simulink library "lib_TCML"  (R2015a)
settings: Solver=ode45  StartTime=0.0  StopTime=10.0  RelTol=1e-3
libraries: simulink x5
(part 5 of 7)

== system lib_TCML/Dynamic Tip Clearance/Case Deformation/Deformation1/Thermal Expansion 1D Elastic ==
  Previous/Reference Length [Lo] : Inport
  Previous/Reference Temperature [To] : Inport  Port=2
  Current Temperature [Tf] : Inport  Port=3
  Add : Sum  Inputs=+-
  Add1 : Sum
  MATLAB Function : MATLAB Function  TreatAsAtomicUnit=on
  Mass Flow Rate on Inner Surface1 : Constant  Value=TempDependence_M
  Mass Flow Rate on Inner Surface2 : Constant  Value=T_data_M
  Mass Flow Rate on Inner Surface3 : Constant  Value=alpha_data_M
  Mass Flow Rate on Inner Surface4 : Constant  Value=alpha_M
  Mass Flow Rate on Inner Surface6 : Constant  Value=BN_M
  Memory : Memory  X0=zeros(1,7)  InheritSampleTime=on
  Product : Product  Inputs=***
  Switch : Switch  Criteria=u2 > Threshold
  Current Length [L] : Outport
  wires:
  Previous/Reference Length [Lo]/1 -> Product/2, Add1/2, MATLAB Function/3(Lo)
  Previous/Reference Temperature [To]/1 -> MATLAB Function/4(To), Add/2
  Current Temperature [Tf]/1 -> MATLAB Function/5(Tf), Add/1
  Mass Flow Rate on Inner Surface6/1 -> MATLAB Function/7(BN)
  MATLAB Function/1(L) -> Switch/1
  Memory/1 -> MATLAB Function/6(Erro)
  MATLAB Function/2(Err) -> Memory/1
  Mass Flow Rate on Inner Surface1/1 -> Switch/2
  Mass Flow Rate on Inner Surface2/1 -> MATLAB Function/1(T_data)
  Mass Flow Rate on Inner Surface3/1 -> MATLAB Function/2(alpha_data)
  Add/1 -> Product/1
  Mass Flow Rate on Inner Surface4/1 -> Product/3
  Switch/1 -> Current Length [L]/1
  Product/1 -> Add1/1
  Add1/1 -> Switch/3

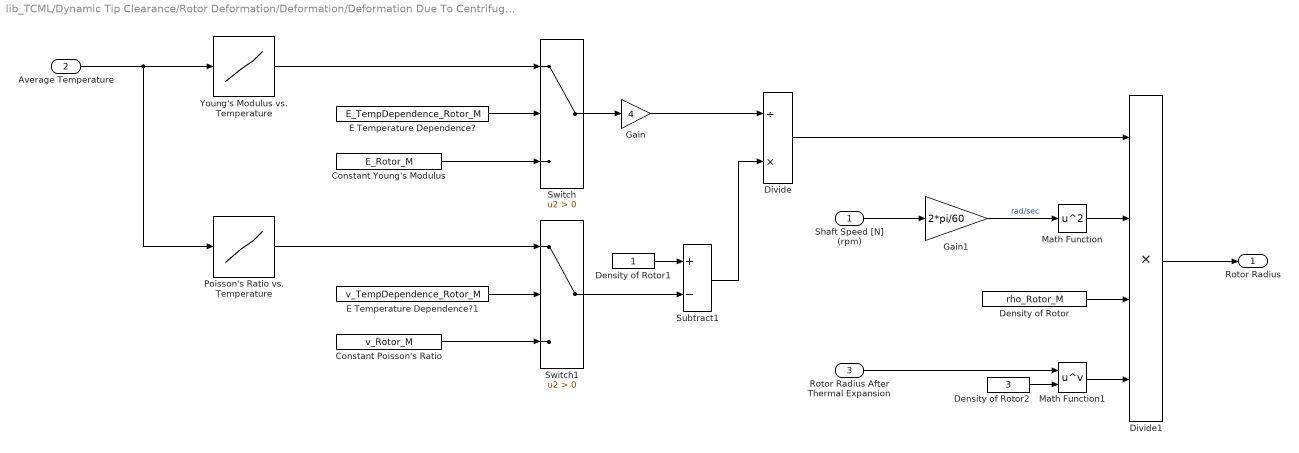
== system lib_TCML/Dynamic Tip Clearance/Rotor Deformation/Deformation/Deformation Due To Centrifugal Forces ==
  Shaft Speed [N] (rpm) : Inport
  Average Temperature : Inport  Port=2
  Rotor Radius After Thermal Expansion : Inport  Port=3
  Constant Poisson's Ratio : Constant  Value=v_Rotor_M
  Constant Young's Modulus : Constant  Value=E_Rotor_M
  Density of Rotor : Constant  Value=rho_Rotor_M
  Density of Rotor1 : Constant
  Density of Rotor2 : Constant  Value=3
  Divide : Product  Inputs=/*
  Divide1 : Product  Inputs=****
  E Temperature Dependence? : Constant  Value=E_TempDependence_Rotor_M
  E Temperature Dependence?1 : Constant  Value=v_TempDependence_Rotor_M
  Gain : Gain  Gain=4
  Gain1 : Gain  Gain=2*pi/60
  Math Function : Math  Operator=square  SaturateOnIntegerOverflow=on
  Math Function1 : Math  Operator=pow  SaturateOnIntegerOverflow=on
  Poisson's Ratio vs. Temperature : Lookup_n-D  NumberOfTableDimensions=1  BreakpointsForDimension1=Tv_Rotor_Data_M  Table=v_Rotor_Data_M  InternalRulePriority=Speed  RndMeth=Simplest  InputSameDT=on
  Subtract1 : Sum  Inputs=+-
  Switch : Switch  Criteria=u2 > Threshold
  Switch1 : Switch  Criteria=u2 > Threshold
  Young's Modulus vs. Temperature : Lookup_n-D  NumberOfTableDimensions=1  BreakpointsForDimension1=TE_Rotor_Data_M  Table=E_Rotor_Data_M  InternalRulePriority=Speed  RndMeth=Simplest  InputSameDT=on
  Rotor Radius : Outport
  wires:
  Constant Poisson's Ratio/1 -> Switch1/3
  Young's Modulus vs. Temperature/1 -> Switch/1
  Poisson's Ratio vs. Temperature/1 -> Switch1/1
  E Temperature Dependence?1/1 -> Switch1/2
  Switch/1 -> Gain/1
  Density of Rotor1/1 -> Subtract1/1
  Constant Young's Modulus/1 -> Switch/3
  Divide/1 -> Divide1/1
  Switch1/1 -> Subtract1/2
  Subtract1/1 -> Divide/2
  Gain/1 -> Divide/1
  Gain1/1 -> Math Function/1  "rad/sec"
  Density of Rotor/1 -> Divide1/3
  E Temperature Dependence?/1 -> Switch/2
  Math Function1/1 -> Divide1/4
  Math Function/1 -> Divide1/2
  Shaft Speed [N] (rpm)/1 -> Gain1/1
  Divide1/1 -> Rotor Radius/1
  Density of Rotor2/1 -> Math Function1/2
  Average Temperature/1 -> Poisson's Ratio vs. Temperature/1, Young's Modulus vs. Temperature/1
  Rotor Radius After Thermal Expansion/1 -> Math Function1/1

== system lib_TCML/Dynamic Tip Clearance/Rotor Deformation/Deformation/Deformation Due To Thermal Expansion ==
  Average Rotor Temperature : Inport
  Memory1 : Memory  X0=mean(T0_Rotor_M)
  Memory2 : Memory  X0=Ro_Rotor_M
  Thermal Expansion 1D Elastic : Subsystem  mask(TSAT: Thermal Expansion Library Block){TempDependence_M=on, alpha_M=alpha_Rotor_M, T_data_M=Talpha_Rotor_Data_M, alpha_data_M=alpha_Rotor_Data_M, BN_M=double(gcb)}
      mask prompts: TempDependence_M "TempDependence_M - Temperature dependence of the thermal expansion coefficient (unchecked - constant, checked - temperature dependent)"; alpha_M "alpha_M - Constant thermal expansion coefficient"; T_data_M "T_data_M - Temperature array (nx1)"; alpha_data_M "alpha_data_M - Thermal expansion coefficient array (nx1)"; BN_M "Block Name"
      mask help:
      | This function calculates the length or radius of a structure that has expanded or contracted due to thermal expansion. The block accepts the previous/reference length (Lo), previous/reference temperature (To), and current temperature (Tf) as its inputs. The user has the option to specify a constant thermal expansion coefficient or to incorporate temperature dependence by providing data that correlates the thermal expansion coefficient with temperature.
      |
      | This block is capable of accepting various units but it is important that the units be consistent across all inputs and parameters. For details on this block, see the block help menu.
      mask init:
      | %set default parameters if they are not being used
      | if TempDependence_M == 0
      |     T_data_M = [0 5000];
      |     alpha_data_M = [10e-6 10e-6];
      | elseif TempDependence_M == 1
      |     alpha_M = 10e-6;
      | end
      mask Help: web(which('Deformation_TSAT_ThermExp1DElastic.html'),'-helpbrowser')
      mask Callback TempDependence_M:
      | MSK_SEC_Enables_TSAT('TempDependence_M',2,'dis')
      | MSK_SEC_Enables_TSAT('TempDependence_M',[3 4],'en')
  Rotor Radius after Thermal Expansion : Outport
  wires:
  Average Rotor Temperature/1 -> Thermal Expansion 1D Elastic/3(Current Temperature [Tf]), Memory1/1
  Memory2/1 -> Thermal Expansion 1D Elastic/1(Previous/Reference Length [Lo])
  Memory1/1 -> Thermal Expansion 1D Elastic/2(Previous/Reference Temperature [To])
  Thermal Expansion 1D Elastic/1(Current Length [L]) -> Memory2/1, Rotor Radius after Thermal Expansion/1

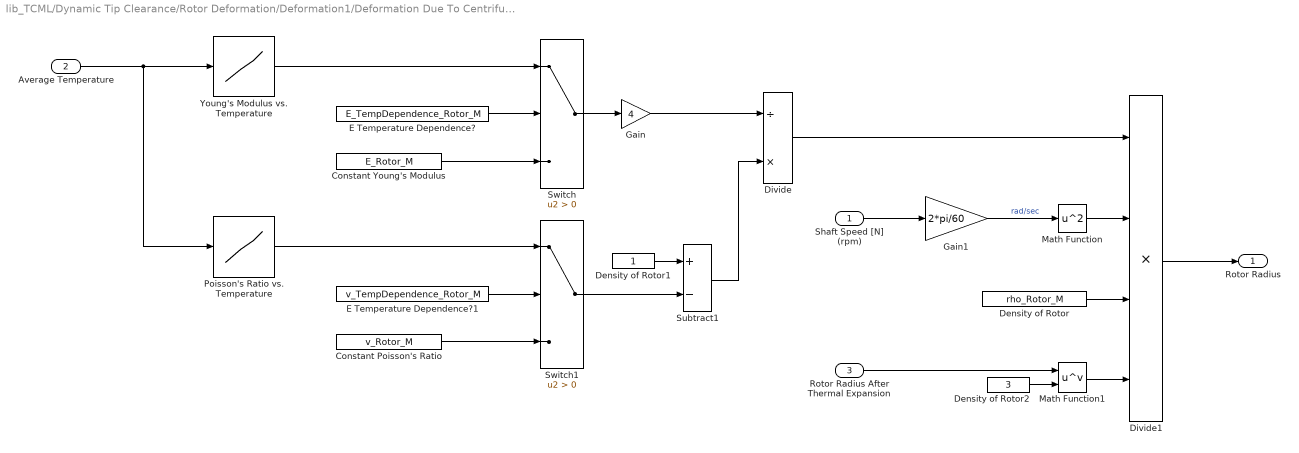
== system lib_TCML/Dynamic Tip Clearance/Rotor Deformation/Deformation1/Deformation Due To Centrifugal Forces ==
  Shaft Speed [N] (rpm) : Inport
  Average Temperature : Inport  Port=2
  Rotor Radius After Thermal Expansion : Inport  Port=3
  Constant Poisson's Ratio : Constant  Value=v_Rotor_M
  Constant Young's Modulus : Constant  Value=E_Rotor_M
  Density of Rotor : Constant  Value=rho_Rotor_M
  Density of Rotor1 : Constant
  Density of Rotor2 : Constant  Value=3
  Divide : Product  Inputs=/*
  Divide1 : Product  Inputs=****
  E Temperature Dependence? : Constant  Value=E_TempDependence_Rotor_M
  E Temperature Dependence?1 : Constant  Value=v_TempDependence_Rotor_M
  Gain : Gain  Gain=4
  Gain1 : Gain  Gain=2*pi/60
  Math Function : Math  Operator=square  SaturateOnIntegerOverflow=on
  Math Function1 : Math  Operator=pow  SaturateOnIntegerOverflow=on
  Poisson's Ratio vs. Temperature : Lookup_n-D  NumberOfTableDimensions=1  BreakpointsForDimension1=Tv_Rotor_Data_M  Table=v_Rotor_Data_M  InternalRulePriority=Speed  RndMeth=Simplest  InputSameDT=on
  Subtract1 : Sum  Inputs=+-
  Switch : Switch  Criteria=u2 > Threshold
  Switch1 : Switch  Criteria=u2 > Threshold
  Young's Modulus vs. Temperature : Lookup_n-D  NumberOfTableDimensions=1  BreakpointsForDimension1=TE_Rotor_Data_M  Table=E_Rotor_Data_M  InternalRulePriority=Speed  RndMeth=Simplest  InputSameDT=on
  Rotor Radius : Outport
  wires:
  Rotor Radius After Thermal Expansion/1 -> Math Function1/1
  Average Temperature/1 -> Young's Modulus vs. Temperature/1, Poisson's Ratio vs. Temperature/1
  Density of Rotor2/1 -> Math Function1/2
  Divide1/1 -> Rotor Radius/1
  Shaft Speed [N] (rpm)/1 -> Gain1/1
  Math Function/1 -> Divide1/2
  Math Function1/1 -> Divide1/4
  E Temperature Dependence?/1 -> Switch/2
  Density of Rotor/1 -> Divide1/3
  Gain1/1 -> Math Function/1  "rad/sec"
  Gain/1 -> Divide/1
  Subtract1/1 -> Divide/2
  Switch1/1 -> Subtract1/2
  Divide/1 -> Divide1/1
  Constant Young's Modulus/1 -> Switch/3
  Density of Rotor1/1 -> Subtract1/1
  Switch/1 -> Gain/1
  E Temperature Dependence?1/1 -> Switch1/2
  Poisson's Ratio vs. Temperature/1 -> Switch1/1
  Young's Modulus vs. Temperature/1 -> Switch/1
  Constant Poisson's Ratio/1 -> Switch1/3

== system lib_TCML/Dynamic Tip Clearance/Rotor Deformation/Deformation1/Deformation Due To Thermal Expansion ==
  Average Rotor Temperature : Inport
  Memory1 : Memory  X0=mean(T0_Rotor_M)
  Memory2 : Memory  X0=Ro_Rotor_M
  Thermal Expansion 1D Elastic : Subsystem  mask(TSAT: Thermal Expansion Library Block){TempDependence_M=on, alpha_M=alpha_Rotor_M, T_data_M=Talpha_Rotor_Data_M, alpha_data_M=alpha_Rotor_Data_M, BN_M=double(gcb)}
      mask prompts: TempDependence_M "TempDependence_M - Temperature dependence of the thermal expansion coefficient (unchecked - constant, checked - temperature dependent)"; alpha_M "alpha_M - Constant thermal expansion coefficient"; T_data_M "T_data_M - Temperature array (nx1)"; alpha_data_M "alpha_data_M - Thermal expansion coefficient array (nx1)"; BN_M "Block Name"
      mask help:
      | This function calculates the length or radius of a structure that has expanded or contracted due to thermal expansion. The block accepts the previous/reference length (Lo), previous/reference temperature (To), and current temperature (Tf) as its inputs. The user has the option to specify a constant thermal expansion coefficient or to incorporate temperature dependence by providing data that correlates the thermal expansion coefficient with temperature.
      |
      | This block is capable of accepting various units but it is important that the units be consistent across all inputs and parameters. For details on this block, see the block help menu.
      mask init:
      | %set default parameters if they are not being used
      | if TempDependence_M == 0
      |     T_data_M = [0 5000];
      |     alpha_data_M = [10e-6 10e-6];
      | elseif TempDependence_M == 1
      |     alpha_M = 10e-6;
      | end
      mask Help: web(which('Deformation_TSAT_ThermExp1DElastic.html'),'-helpbrowser')
      mask Callback TempDependence_M:
      | MSK_SEC_Enables_TSAT('TempDependence_M',2,'dis')
      | MSK_SEC_Enables_TSAT('TempDependence_M',[3 4],'en')
  Rotor Radius after Thermal Expansion : Outport
  wires:
  Thermal Expansion 1D Elastic/1(Current Length [L]) -> Rotor Radius after Thermal Expansion/1, Memory2/1
  Memory1/1 -> Thermal Expansion 1D Elastic/2(Previous/Reference Temperature [To])
  Memory2/1 -> Thermal Expansion 1D Elastic/1(Previous/Reference Length [Lo])
  Average Rotor Temperature/1 -> Memory1/1, Thermal Expansion 1D Elastic/3(Current Temperature [Tf])

== system lib_TCML/Steady-State Tip Clearance/Blade Deformation/Deformation/Deformation Due To Centrifugal Forces ==
  Shaft Speed [N] (rpm) : Inport
  Average Temperature : Inport  Port=2
  Blade Length After Thermal Expansion : Inport  Port=3
  Rotor Outer Radius : Inport  Port=4
  Add : Sum
  Constant Young's Modulus : Constant  Value=E_Blade_M
  Density of Rotor : Constant  Value=rho_Blade_M
  Density of Rotor1 : Constant
  Divide : Product  Inputs=/*
  Divide1 : Product  Inputs=****
  Divide2 : Product  Inputs=**
  E Temperature Dependence? : Constant  Value=E_TempDependence_Blade_M
  Gain1 : Gain  Gain=2*pi/60
  Math Function : Math  Operator=square  SaturateOnIntegerOverflow=on
  Math Function2 : Math  Operator=square  SaturateOnIntegerOverflow=on
  Switch : Switch  Criteria=u2 > Threshold
  Young's Modulus vs. Temperature : Lookup_n-D  NumberOfTableDimensions=1  BreakpointsForDimension1=TE_Blade_Data_M  Table=E_Blade_Data_M  InternalRulePriority=Speed  RndMeth=Simplest  InputSameDT=on
  Blade Length : Outport
  wires:
  Young's Modulus vs. Temperature/1 -> Switch/1
  Density of Rotor1/1 -> Divide/2
  Constant Young's Modulus/1 -> Switch/3
  Divide/1 -> Divide1/1
  Switch/1 -> Divide/1
  Gain1/1 -> Math Function/1  "rad/sec"
  Density of Rotor/1 -> Divide1/3
  E Temperature Dependence?/1 -> Switch/2
  Math Function/1 -> Divide1/2
  Shaft Speed [N] (rpm)/1 -> Gain1/1
  Divide1/1 -> Blade Length/1
  Average Temperature/1 -> Young's Modulus vs. Temperature/1
  Blade Length After Thermal Expansion/1 -> Add/2, Math Function2/1
  Rotor Outer Radius/1 -> Add/1
  Add/1 -> Divide2/1
  Math Function2/1 -> Divide2/2
  Divide2/1 -> Divide1/4

== system lib_TCML/Steady-State Tip Clearance/Blade Deformation/Deformation/Deformation Due To Thermal Expansion ==
  Average Rotor Temperature : Inport
  Memory1 : Memory  X0=T0_Blade_M
  Memory2 : Memory  X0=L_Blade_M
  Thermal Expansion 1D Elastic : Subsystem  mask(TSAT: Thermal Expansion Library Block){TempDependence_M=on, alpha_M=alpha_Blade_M, T_data_M=Talpha_Blade_Data_M, alpha_data_M=alpha_Blade_Data_M, BN_M=double(gcb)}
      mask prompts: TempDependence_M "TempDependence_M - Temperature dependence of the thermal expansion coefficient (unchecked - constant, checked - temperature dependent)"; alpha_M "alpha_M - Constant thermal expansion coefficient"; T_data_M "T_data_M - Temperature array (nx1)"; alpha_data_M "alpha_data_M - Thermal expansion coefficient array (nx1)"; BN_M "Block Name"
      mask help:
      | This function calculates the length or radius of a structure that has expanded or contracted due to thermal expansion. The block accepts the previous/reference length (Lo), previous/reference temperature (To), and current temperature (Tf) as its inputs. The user has the option to specify a constant thermal expansion coefficient or to incorporate temperature dependence by providing data that correlates the thermal expansion coefficient with temperature.
      |
      | This block is capable of accepting various units but it is important that the units be consistent across all inputs and parameters. For details on this block, see the block help menu.
      mask init:
      | %set default parameters if they are not being used
      | if TempDependence_M == 0
      |     T_data_M = [0 5000];
      |     alpha_data_M = [10e-6 10e-6];
      | elseif TempDependence_M == 1
      |     alpha_M = 10e-6;
      | end
      mask Help: web(which('Deformation_TSAT_ThermExp1DElastic.html'),'-helpbrowser')
      mask Callback TempDependence_M:
      | MSK_SEC_Enables_TSAT('TempDependence_M',2,'dis')
      | MSK_SEC_Enables_TSAT('TempDependence_M',[3 4],'en')
  Blade Length after Thermal Expansion : Outport
  wires:
  Average Rotor Temperature/1 -> Thermal Expansion 1D Elastic/3(Current Temperature [Tf]), Memory1/1
  Memory2/1 -> Thermal Expansion 1D Elastic/1(Previous/Reference Length [Lo])
  Memory1/1 -> Thermal Expansion 1D Elastic/2(Previous/Reference Temperature [To])
  Thermal Expansion 1D Elastic/1(Current Length [L]) -> Memory2/1, Blade Length after Thermal Expansion/1

== system lib_TCML/Steady-State Tip Clearance/Case Deformation/Deformation/Thermal Expansion 1D Elastic ==
  Previous/Reference Length [Lo] : Inport
  Previous/Reference Temperature [To] : Inport  Port=2
  Current Temperature [Tf] : Inport  Port=3
  Add : Sum  Inputs=+-
  Add1 : Sum
  MATLAB Function : MATLAB Function  TreatAsAtomicUnit=on
  Mass Flow Rate on Inner Surface1 : Constant  Value=TempDependence_M
  Mass Flow Rate on Inner Surface2 : Constant  Value=T_data_M
  Mass Flow Rate on Inner Surface3 : Constant  Value=alpha_data_M
  Mass Flow Rate on Inner Surface4 : Constant  Value=alpha_M
  Mass Flow Rate on Inner Surface6 : Constant  Value=BN_M
  Memory : Memory  X0=zeros(1,7)  InheritSampleTime=on
  Product : Product  Inputs=***
  Switch : Switch  Criteria=u2 > Threshold
  Current Length [L] : Outport
  wires:
  Previous/Reference Length [Lo]/1 -> Product/2, Add1/2, MATLAB Function/3(Lo)
  Previous/Reference Temperature [To]/1 -> MATLAB Function/4(To), Add/2
  Current Temperature [Tf]/1 -> MATLAB Function/5(Tf), Add/1
  Mass Flow Rate on Inner Surface6/1 -> MATLAB Function/7(BN)
  MATLAB Function/1(L) -> Switch/1
  Memory/1 -> MATLAB Function/6(Erro)
  MATLAB Function/2(Err) -> Memory/1
  Mass Flow Rate on Inner Surface1/1 -> Switch/2
  Mass Flow Rate on Inner Surface2/1 -> MATLAB Function/1(T_data)
  Mass Flow Rate on Inner Surface3/1 -> MATLAB Function/2(alpha_data)
  Add/1 -> Product/1
  Mass Flow Rate on Inner Surface4/1 -> Product/3
  Switch/1 -> Current Length [L]/1
  Product/1 -> Add1/1
  Add1/1 -> Switch/3

== system lib_TCML/Steady-State Tip Clearance/Case Deformation/Deformation1/Thermal Expansion 1D Elastic ==
  Previous/Reference Length [Lo] : Inport
  Previous/Reference Temperature [To] : Inport  Port=2
  Current Temperature [Tf] : Inport  Port=3
  Add : Sum  Inputs=+-
  Add1 : Sum
  MATLAB Function : MATLAB Function  TreatAsAtomicUnit=on
  Mass Flow Rate on Inner Surface1 : Constant  Value=TempDependence_M
  Mass Flow Rate on Inner Surface2 : Constant  Value=T_data_M
  Mass Flow Rate on Inner Surface3 : Constant  Value=alpha_data_M
  Mass Flow Rate on Inner Surface4 : Constant  Value=alpha_M
  Mass Flow Rate on Inner Surface6 : Constant  Value=BN_M
  Memory : Memory  X0=zeros(1,7)  InheritSampleTime=on
  Product : Product  Inputs=***
  Switch : Switch  Criteria=u2 > Threshold
  Current Length [L] : Outport
  wires:
  Add1/1 -> Switch/3
  Product/1 -> Add1/1
  Switch/1 -> Current Length [L]/1
  Mass Flow Rate on Inner Surface4/1 -> Product/3
  Add/1 -> Product/1
  Mass Flow Rate on Inner Surface3/1 -> MATLAB Function/2(alpha_data)
  Mass Flow Rate on Inner Surface2/1 -> MATLAB Function/1(T_data)
  Mass Flow Rate on Inner Surface1/1 -> Switch/2
  MATLAB Function/2(Err) -> Memory/1
  Memory/1 -> MATLAB Function/6(Erro)
  MATLAB Function/1(L) -> Switch/1
  Mass Flow Rate on Inner Surface6/1 -> MATLAB Function/7(BN)
  Current Temperature [Tf]/1 -> Add/1, MATLAB Function/5(Tf)
  Previous/Reference Temperature [To]/1 -> Add/2, MATLAB Function/4(To)
  Previous/Reference Length [Lo]/1 -> MATLAB Function/3(Lo), Add1/2, Product/2

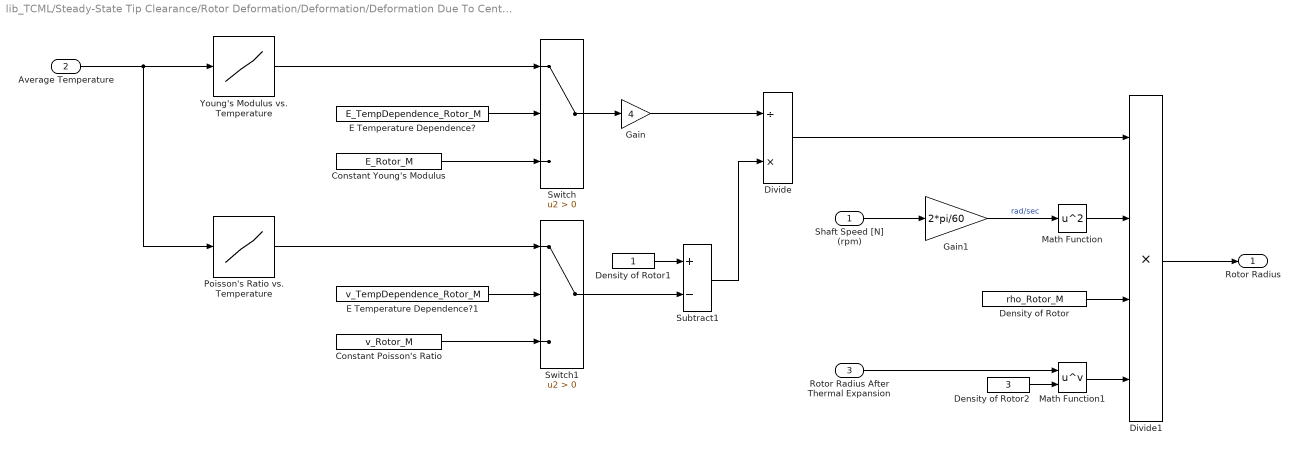
== system lib_TCML/Steady-State Tip Clearance/Rotor Deformation/Deformation/Deformation Due To Centrifugal Forces ==
  Shaft Speed [N] (rpm) : Inport
  Average Temperature : Inport  Port=2
  Rotor Radius After Thermal Expansion : Inport  Port=3
  Constant Poisson's Ratio : Constant  Value=v_Rotor_M
  Constant Young's Modulus : Constant  Value=E_Rotor_M
  Density of Rotor : Constant  Value=rho_Rotor_M
  Density of Rotor1 : Constant
  Density of Rotor2 : Constant  Value=3
  Divide : Product  Inputs=/*
  Divide1 : Product  Inputs=****
  E Temperature Dependence? : Constant  Value=E_TempDependence_Rotor_M
  E Temperature Dependence?1 : Constant  Value=v_TempDependence_Rotor_M
  Gain : Gain  Gain=4
  Gain1 : Gain  Gain=2*pi/60
  Math Function : Math  Operator=square  SaturateOnIntegerOverflow=on
  Math Function1 : Math  Operator=pow  SaturateOnIntegerOverflow=on
  Poisson's Ratio vs. Temperature : Lookup_n-D  NumberOfTableDimensions=1  BreakpointsForDimension1=Tv_Rotor_Data_M  Table=v_Rotor_Data_M  InternalRulePriority=Speed  RndMeth=Simplest  InputSameDT=on
  Subtract1 : Sum  Inputs=+-
  Switch : Switch  Criteria=u2 > Threshold
  Switch1 : Switch  Criteria=u2 > Threshold
  Young's Modulus vs. Temperature : Lookup_n-D  NumberOfTableDimensions=1  BreakpointsForDimension1=TE_Rotor_Data_M  Table=E_Rotor_Data_M  InternalRulePriority=Speed  RndMeth=Simplest  InputSameDT=on
  Rotor Radius : Outport
  wires:
  Constant Poisson's Ratio/1 -> Switch1/3
  Young's Modulus vs. Temperature/1 -> Switch/1
  Poisson's Ratio vs. Temperature/1 -> Switch1/1
  E Temperature Dependence?1/1 -> Switch1/2
  Switch/1 -> Gain/1
  Density of Rotor1/1 -> Subtract1/1
  Constant Young's Modulus/1 -> Switch/3
  Divide/1 -> Divide1/1
  Switch1/1 -> Subtract1/2
  Subtract1/1 -> Divide/2
  Gain/1 -> Divide/1
  Gain1/1 -> Math Function/1  "rad/sec"
  Density of Rotor/1 -> Divide1/3
  E Temperature Dependence?/1 -> Switch/2
  Math Function1/1 -> Divide1/4
  Math Function/1 -> Divide1/2
  Shaft Speed [N] (rpm)/1 -> Gain1/1
  Divide1/1 -> Rotor Radius/1
  Density of Rotor2/1 -> Math Function1/2
  Average Temperature/1 -> Poisson's Ratio vs. Temperature/1, Young's Modulus vs. Temperature/1
  Rotor Radius After Thermal Expansion/1 -> Math Function1/1

== system lib_TCML/Steady-State Tip Clearance/Rotor Deformation/Deformation/Deformation Due To Thermal Expansion ==
  Average Rotor Temperature : Inport
  Memory1 : Memory  X0=mean(T0_Rotor_M)
  Memory2 : Memory  X0=Ro_Rotor_M
  Thermal Expansion 1D Elastic : Subsystem  mask(TSAT: Thermal Expansion Library Block){TempDependence_M=on, alpha_M=alpha_Rotor_M, T_data_M=Talpha_Rotor_Data_M, alpha_data_M=alpha_Rotor_Data_M, BN_M=double(gcb)}
      mask prompts: TempDependence_M "TempDependence_M - Temperature dependence of the thermal expansion coefficient (unchecked - constant, checked - temperature dependent)"; alpha_M "alpha_M - Constant thermal expansion coefficient"; T_data_M "T_data_M - Temperature array (nx1)"; alpha_data_M "alpha_data_M - Thermal expansion coefficient array (nx1)"; BN_M "Block Name"
      mask help:
      | This function calculates the length or radius of a structure that has expanded or contracted due to thermal expansion. The block accepts the previous/reference length (Lo), previous/reference temperature (To), and current temperature (Tf) as its inputs. The user has the option to specify a constant thermal expansion coefficient or to incorporate temperature dependence by providing data that correlates the thermal expansion coefficient with temperature.
      |
      | This block is capable of accepting various units but it is important that the units be consistent across all inputs and parameters. For details on this block, see the block help menu.
      mask init:
      | %set default parameters if they are not being used
      | if TempDependence_M == 0
      |     T_data_M = [0 5000];
      |     alpha_data_M = [10e-6 10e-6];
      | elseif TempDependence_M == 1
      |     alpha_M = 10e-6;
      | end
      mask Help: web(which('Deformation_TSAT_ThermExp1DElastic.html'),'-helpbrowser')
      mask Callback TempDependence_M:
      | MSK_SEC_Enables_TSAT('TempDependence_M',2,'dis')
      | MSK_SEC_Enables_TSAT('TempDependence_M',[3 4],'en')
  Rotor Radius after Thermal Expansion : Outport
  wires:
  Average Rotor Temperature/1 -> Thermal Expansion 1D Elastic/3(Current Temperature [Tf]), Memory1/1
  Memory2/1 -> Thermal Expansion 1D Elastic/1(Previous/Reference Length [Lo])
  Memory1/1 -> Thermal Expansion 1D Elastic/2(Previous/Reference Temperature [To])
  Thermal Expansion 1D Elastic/1(Current Length [L]) -> Memory2/1, Rotor Radius after Thermal Expansion/1

== system lib_TCML/Dynamic Tip Clearance/Blade Deformation/Deformation/Deformation Due To Thermal Expansion/Thermal Expansion 1D Elastic ==
  Previous/Reference Length [Lo] : Inport
  Previous/Reference Temperature [To] : Inport  Port=2
  Current Temperature [Tf] : Inport  Port=3
  Add : Sum  Inputs=+-
  Add1 : Sum
  MATLAB Function : MATLAB Function  TreatAsAtomicUnit=on
  Mass Flow Rate on Inner Surface1 : Constant  Value=TempDependence_M
  Mass Flow Rate on Inner Surface2 : Constant  Value=T_data_M
  Mass Flow Rate on Inner Surface3 : Constant  Value=alpha_data_M
  Mass Flow Rate on Inner Surface4 : Constant  Value=alpha_M
  Mass Flow Rate on Inner Surface6 : Constant  Value=BN_M
  Memory : Memory  X0=zeros(1,7)  InheritSampleTime=on
  Product : Product  Inputs=***
  Switch : Switch  Criteria=u2 > Threshold
  Current Length [L] : Outport
  wires:
  Previous/Reference Length [Lo]/1 -> Product/2, Add1/2, MATLAB Function/3(Lo)
  Previous/Reference Temperature [To]/1 -> MATLAB Function/4(To), Add/2
  Current Temperature [Tf]/1 -> MATLAB Function/5(Tf), Add/1
  Mass Flow Rate on Inner Surface6/1 -> MATLAB Function/7(BN)
  MATLAB Function/1(L) -> Switch/1
  Memory/1 -> MATLAB Function/6(Erro)
  MATLAB Function/2(Err) -> Memory/1
  Mass Flow Rate on Inner Surface1/1 -> Switch/2
  Mass Flow Rate on Inner Surface2/1 -> MATLAB Function/1(T_data)
  Mass Flow Rate on Inner Surface3/1 -> MATLAB Function/2(alpha_data)
  Add/1 -> Product/1
  Mass Flow Rate on Inner Surface4/1 -> Product/3
  Switch/1 -> Current Length [L]/1
  Product/1 -> Add1/1
  Add1/1 -> Switch/3

== system lib_TCML/Dynamic Tip Clearance/Blade Deformation/Deformation1/Deformation Due To Thermal Expansion/Thermal Expansion 1D Elastic ==
  Previous/Reference Length [Lo] : Inport
  Previous/Reference Temperature [To] : Inport  Port=2
  Current Temperature [Tf] : Inport  Port=3
  Add : Sum  Inputs=+-
  Add1 : Sum
  MATLAB Function : MATLAB Function  TreatAsAtomicUnit=on
  Mass Flow Rate on Inner Surface1 : Constant  Value=TempDependence_M
  Mass Flow Rate on Inner Surface2 : Constant  Value=T_data_M
  Mass Flow Rate on Inner Surface3 : Constant  Value=alpha_data_M
  Mass Flow Rate on Inner Surface4 : Constant  Value=alpha_M
  Mass Flow Rate on Inner Surface6 : Constant  Value=BN_M
  Memory : Memory  X0=zeros(1,7)  InheritSampleTime=on
  Product : Product  Inputs=***
  Switch : Switch  Criteria=u2 > Threshold
  Current Length [L] : Outport
  wires:
  Previous/Reference Length [Lo]/1 -> Product/2, Add1/2, MATLAB Function/3(Lo)
  Previous/Reference Temperature [To]/1 -> MATLAB Function/4(To), Add/2
  Current Temperature [Tf]/1 -> MATLAB Function/5(Tf), Add/1
  Mass Flow Rate on Inner Surface6/1 -> MATLAB Function/7(BN)
  MATLAB Function/1(L) -> Switch/1
  Memory/1 -> MATLAB Function/6(Erro)
  MATLAB Function/2(Err) -> Memory/1
  Mass Flow Rate on Inner Surface1/1 -> Switch/2
  Mass Flow Rate on Inner Surface2/1 -> MATLAB Function/1(T_data)
  Mass Flow Rate on Inner Surface3/1 -> MATLAB Function/2(alpha_data)
  Add/1 -> Product/1
  Mass Flow Rate on Inner Surface4/1 -> Product/3
  Switch/1 -> Current Length [L]/1
  Product/1 -> Add1/1
  Add1/1 -> Switch/3

== system lib_TCML/Dynamic Tip Clearance/Rotor Deformation/Deformation/Deformation Due To Thermal Expansion/Thermal Expansion 1D Elastic ==
  Previous/Reference Length [Lo] : Inport
  Previous/Reference Temperature [To] : Inport  Port=2
  Current Temperature [Tf] : Inport  Port=3
  Add : Sum  Inputs=+-
  Add1 : Sum
  MATLAB Function : MATLAB Function  TreatAsAtomicUnit=on
  Mass Flow Rate on Inner Surface1 : Constant  Value=TempDependence_M
  Mass Flow Rate on Inner Surface2 : Constant  Value=T_data_M
  Mass Flow Rate on Inner Surface3 : Constant  Value=alpha_data_M
  Mass Flow Rate on Inner Surface4 : Constant  Value=alpha_M
  Mass Flow Rate on Inner Surface6 : Constant  Value=BN_M
  Memory : Memory  X0=zeros(1,7)  InheritSampleTime=on
  Product : Product  Inputs=***
  Switch : Switch  Criteria=u2 > Threshold
  Current Length [L] : Outport
  wires:
  Previous/Reference Length [Lo]/1 -> Product/2, Add1/2, MATLAB Function/3(Lo)
  Previous/Reference Temperature [To]/1 -> MATLAB Function/4(To), Add/2
  Current Temperature [Tf]/1 -> MATLAB Function/5(Tf), Add/1
  Mass Flow Rate on Inner Surface6/1 -> MATLAB Function/7(BN)
  MATLAB Function/1(L) -> Switch/1
  Memory/1 -> MATLAB Function/6(Erro)
  MATLAB Function/2(Err) -> Memory/1
  Mass Flow Rate on Inner Surface1/1 -> Switch/2
  Mass Flow Rate on Inner Surface2/1 -> MATLAB Function/1(T_data)
  Mass Flow Rate on Inner Surface3/1 -> MATLAB Function/2(alpha_data)
  Add/1 -> Product/1
  Mass Flow Rate on Inner Surface4/1 -> Product/3
  Switch/1 -> Current Length [L]/1
  Product/1 -> Add1/1
  Add1/1 -> Switch/3

== system lib_TCML/Dynamic Tip Clearance/Rotor Deformation/Deformation1/Deformation Due To Thermal Expansion/Thermal Expansion 1D Elastic ==
  Previous/Reference Length [Lo] : Inport
  Previous/Reference Temperature [To] : Inport  Port=2
  Current Temperature [Tf] : Inport  Port=3
  Add : Sum  Inputs=+-
  Add1 : Sum
  MATLAB Function : MATLAB Function  TreatAsAtomicUnit=on
  Mass Flow Rate on Inner Surface1 : Constant  Value=TempDependence_M
  Mass Flow Rate on Inner Surface2 : Constant  Value=T_data_M
  Mass Flow Rate on Inner Surface3 : Constant  Value=alpha_data_M
  Mass Flow Rate on Inner Surface4 : Constant  Value=alpha_M
  Mass Flow Rate on Inner Surface6 : Constant  Value=BN_M
  Memory : Memory  X0=zeros(1,7)  InheritSampleTime=on
  Product : Product  Inputs=***
  Switch : Switch  Criteria=u2 > Threshold
  Current Length [L] : Outport
  wires:
  Previous/Reference Length [Lo]/1 -> Product/2, Add1/2, MATLAB Function/3(Lo)
  Previous/Reference Temperature [To]/1 -> MATLAB Function/4(To), Add/2
  Current Temperature [Tf]/1 -> MATLAB Function/5(Tf), Add/1
  Mass Flow Rate on Inner Surface6/1 -> MATLAB Function/7(BN)
  MATLAB Function/1(L) -> Switch/1
  Memory/1 -> MATLAB Function/6(Erro)
  MATLAB Function/2(Err) -> Memory/1
  Mass Flow Rate on Inner Surface1/1 -> Switch/2
  Mass Flow Rate on Inner Surface2/1 -> MATLAB Function/1(T_data)
  Mass Flow Rate on Inner Surface3/1 -> MATLAB Function/2(alpha_data)
  Add/1 -> Product/1
  Mass Flow Rate on Inner Surface4/1 -> Product/3
  Switch/1 -> Current Length [L]/1
  Product/1 -> Add1/1
  Add1/1 -> Switch/3

== system lib_TCML/Steady-State Tip Clearance/Blade Deformation/Deformation/Deformation Due To Thermal Expansion/Thermal Expansion 1D Elastic ==
  Previous/Reference Length [Lo] : Inport
  Previous/Reference Temperature [To] : Inport  Port=2
  Current Temperature [Tf] : Inport  Port=3
  Add : Sum  Inputs=+-
  Add1 : Sum
  MATLAB Function : MATLAB Function  TreatAsAtomicUnit=on
  Mass Flow Rate on Inner Surface1 : Constant  Value=TempDependence_M
  Mass Flow Rate on Inner Surface2 : Constant  Value=T_data_M
  Mass Flow Rate on Inner Surface3 : Constant  Value=alpha_data_M
  Mass Flow Rate on Inner Surface4 : Constant  Value=alpha_M
  Mass Flow Rate on Inner Surface6 : Constant  Value=BN_M
  Memory : Memory  X0=zeros(1,7)  InheritSampleTime=on
  Product : Product  Inputs=***
  Switch : Switch  Criteria=u2 > Threshold
  Current Length [L] : Outport
  wires:
  Previous/Reference Length [Lo]/1 -> Product/2, Add1/2, MATLAB Function/3(Lo)
  Previous/Reference Temperature [To]/1 -> MATLAB Function/4(To), Add/2
  Current Temperature [Tf]/1 -> MATLAB Function/5(Tf), Add/1
  Mass Flow Rate on Inner Surface6/1 -> MATLAB Function/7(BN)
  MATLAB Function/1(L) -> Switch/1
  Memory/1 -> MATLAB Function/6(Erro)
  MATLAB Function/2(Err) -> Memory/1
  Mass Flow Rate on Inner Surface1/1 -> Switch/2
  Mass Flow Rate on Inner Surface2/1 -> MATLAB Function/1(T_data)
  Mass Flow Rate on Inner Surface3/1 -> MATLAB Function/2(alpha_data)
  Add/1 -> Product/1
  Mass Flow Rate on Inner Surface4/1 -> Product/3
  Switch/1 -> Current Length [L]/1
  Product/1 -> Add1/1
  Add1/1 -> Switch/3

== system lib_TCML/Steady-State Tip Clearance/Rotor Deformation/Deformation/Deformation Due To Thermal Expansion/Thermal Expansion 1D Elastic ==
  Previous/Reference Length [Lo] : Inport
  Previous/Reference Temperature [To] : Inport  Port=2
  Current Temperature [Tf] : Inport  Port=3
  Add : Sum  Inputs=+-
  Add1 : Sum
  MATLAB Function : MATLAB Function  TreatAsAtomicUnit=on
  Mass Flow Rate on Inner Surface1 : Constant  Value=TempDependence_M
  Mass Flow Rate on Inner Surface2 : Constant  Value=T_data_M
  Mass Flow Rate on Inner Surface3 : Constant  Value=alpha_data_M
  Mass Flow Rate on Inner Surface4 : Constant  Value=alpha_M
  Mass Flow Rate on Inner Surface6 : Constant  Value=BN_M
  Memory : Memory  X0=zeros(1,7)  InheritSampleTime=on
  Product : Product  Inputs=***
  Switch : Switch  Criteria=u2 > Threshold
  Current Length [L] : Outport
  wires:
  Previous/Reference Length [Lo]/1 -> Product/2, Add1/2, MATLAB Function/3(Lo)
  Previous/Reference Temperature [To]/1 -> MATLAB Function/4(To), Add/2
  Current Temperature [Tf]/1 -> MATLAB Function/5(Tf), Add/1
  Mass Flow Rate on Inner Surface6/1 -> MATLAB Function/7(BN)
  MATLAB Function/1(L) -> Switch/1
  Memory/1 -> MATLAB Function/6(Erro)
  MATLAB Function/2(Err) -> Memory/1
  Mass Flow Rate on Inner Surface1/1 -> Switch/2
  Mass Flow Rate on Inner Surface2/1 -> MATLAB Function/1(T_data)
  Mass Flow Rate on Inner Surface3/1 -> MATLAB Function/2(alpha_data)
  Add/1 -> Product/1
  Mass Flow Rate on Inner Surface4/1 -> Product/3
  Switch/1 -> Current Length [L]/1
  Product/1 -> Add1/1
  Add1/1 -> Switch/3

== matlab function lib_TCML/Dynamic Tip Clearance/Case Deformation/Deformation/Thermal Expansion 1D Elastic/MATLAB Function ==
  data: T_data input; L output; alpha_data input; Lo input; To input; Tf input; Erro input; BN input; Err output
function [L,Err] = ThermalExpansion(T_data,alpha_data,Lo,To,Tf,Erro,BN)
%#codegen

% initialize error/warning array
Err = Erro;
ErrNum = 1; %Error index

% number of data points for interpolation and numerical integration
n = 50;

%check input sizes
if length(T_data) < 2 && Erro(ErrNum) == 0
    Err(ErrNum) = 1;
    fprintf('warning in %s: The temperature data array (T_data) must be an array of at least 2 elements\n',char(BN));
end
ErrNum = ErrNum + 1;
if length(T_data) ~= length(alpha_data) && Erro(ErrNum) == 0
    Err(ErrNum) = 1;
    fprintf('warning in %s: The temperature data array (T_data) and corresponding thermal expansion coefficient data array (alpha_data) must be the same size\n',char(BN));
end
ErrNum = ErrNum + 1;
    
%check that To and Tf are in the range of T_data
if To < min(T_data)
    To = min(T_data);
    Err(ErrNum) = 1;
    if Erro(ErrNum) == 0
        fprintf('warning in %s: The previous/reference temperature (To) is less than the minimum value of the temperature data array T_data. Expand the data arrays to assure good results. The previous/reference temperature (To) has been set to the minimum value of T_data to avoid errors.\n',char(BN));
    end
end
ErrNum = ErrNum + 1;
if To > max(T_data)
    To = max(T_data);
    Err(ErrNum) = 1;
    if Erro(ErrNum) == 0
        fprintf('warning in %s: The previous/reference temperature (To) is greater than the maximum value of the temperature data array T_data. Expand the data arrays to assure good results. The previous/reference temperature (To) has been set to the maximum value of T_data to avoid errors.\n',char(BN));
    end
end
ErrNum = ErrNum + 1;
if Tf < min(T_data)
    Tf = min(T_data);
    Err(ErrNum) = 1;
    if Erro(ErrNum) == 0
        fprintf('warning in %s: The current temperature (Tf) is less than the minimum value of the temperature data array T_data. Expand the data arrays to assure good results. The current temperature (Tf) has been set to the maximum value of T_data to avoid errors.\n',char(BN));
    end
end
ErrNum = ErrNum + 1;
if Tf > max(T_data)
    Tf = max(T_data);
    Err(ErrNum) = 1;
    if Erro(ErrNum) == 0
        fprintf('warning in %s: The current temperature (Tf) is greater than the maximum value of the temperature data array T_data. Expand the data arrays to assure good results. The current temperature (Tf) has been set to the maximum value of T_data to avoid errors.\n',char(BN));
    end
end
ErrNum = ErrNum + 1;

%check that T_data is monotonically increasing
diffT = diff(T_data);
if min(diffT) <= 0 && Erro(ErrNum) == 0
    Err(ErrNum) = 1;
    fprintf('warning in %s: The temperature data array (T_data) must be monotonically increasing\n',char(BN));
end

T = linspace(To,Tf,n);
alpha = zeros(1,n);
for i = 1:n
    alpha(i) = interp1(T_data,alpha_data,T(i),'linear');
end

Int_alphadT = trapz(T,alpha);
dL = Lo*Int_alphadT;

L = Lo + dL;
